simulink model "rot4b"  (R2015a)
settings: Solver=ode45  StartTime=0.0  StopTime=10.0  RelTol=1e-3
undefined symbols (not defined in the file): L, R, ref, Ts
settings Model: CovSFcnEnable=off  Creator=sebastian  LastModifiedBy=Alexander
settings DebuggingCC: SolverPrmCheckMsg=warning

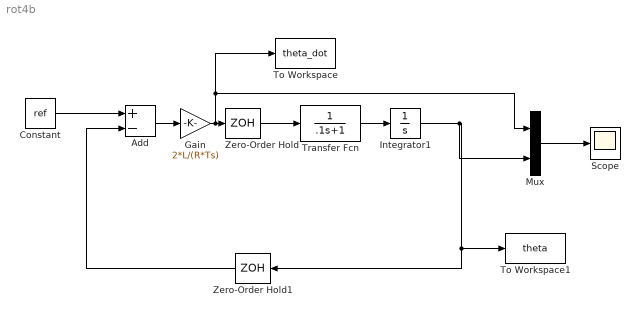
== system rot4b ==
  Add : Sum  Inputs=+-
  Constant : Constant  Value=ref
  Gain : Gain  Gain=2*L/(R*Ts)
  Integrator1 : Integrator  InitialCondition=1
  Mux : Mux  Inputs=2
  Scope : Scope
  To Workspace : ToWorkspace  VariableName=theta_dot  SaveFormat=Timeseries  SampleTime=-1
  To Workspace1 : ToWorkspace  VariableName=theta  SaveFormat=Timeseries  SampleTime=-1
  Transfer Fcn : TransferFcn  Denominator=[.1 1]
  Zero-Order Hold : ZeroOrderHold  SampleTime=Ts
  Zero-Order Hold1 : ZeroOrderHold  SampleTime=Ts
  wires:
  Constant/1 -> Add/1
  Mux/1 -> Scope/1
  Integrator1/1 -> Mux/2, Zero-Order Hold1/1, To Workspace1/1
  Transfer Fcn/1 -> Integrator1/1
  Zero-Order Hold/1 -> Transfer Fcn/1
  Add/1 -> Gain/1
  Gain/1 -> To Workspace/1, Mux/1, Zero-Order Hold/1
  Zero-Order Hold1/1 -> Add/2
